simulink model "test_separator"  (R2021b)
settings: Solver=VariableStepAuto  StartTime=0.0  StopTime=20  RelTol=1e-3
settings Model: Creator=Edwar  LastModifiedBy=Edwar

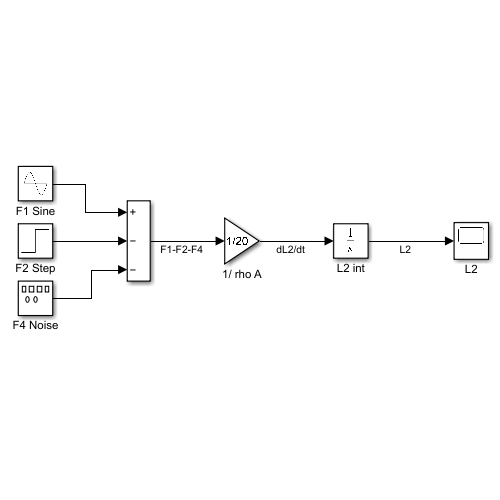
[thumbnail: Simulink's stored preview of the top-level diagram]
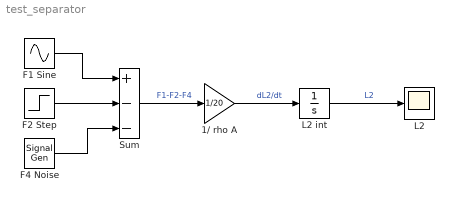
== system test_separator ==
  1/ rho A : Gain  Gain=1/20
  F1 Sine : Sin  SampleTime=0
  F2 Step : Step  SampleTime=0
  F4 Noise : SignalGenerator  Amplitude=10  Frequency=10  Units=rad/sec
  L2 : Scope
  L2 int : Integrator
  Sum : Sum  Inputs=+--
  wires:
  F2 Step/1 -> Sum/2
  F4 Noise/1 -> Sum/3
  F1 Sine/1 -> Sum/1
  Sum/1 -> 1/ rho A/1  "F1-F2-F4"
  1/ rho A/1 -> L2 int/1  "dL2/dt"
  L2 int/1 -> L2/1  "L2"
